simulink model "Schwingungstilger"  (R2024b)
settings: Solver=VariableStepAuto  StartTime=0.0  StopTime=10  RelTol=1e-13  AbsTol=1e-13
values from neighbouring files (symbols this model uses):
  c1 = 100e3    (= 100000)    [Schwingungstilger_Skript.m]    (also in Schwingungstilger_Skript_3d_v2.m; Schwingungstilger_Skript_fminsearch.m; v3_3d_finish.mat; v3_3d_finish_correct.mat)
  c2 = c2_man    (= 3650)    [Schwingungstilger_Skript.m]    (also in Schwingungstilger_Skript_3d_redraw_v2.m = c2_values(cIdx); Schwingungstilger_Skript_3d_v2.m = c2_values(cIdx); Schwingungstilger_Skript_fminsearch.m = params(1); v3_3d_finish.mat = 5000)
  d2 = 15    [Schwingungstilger_Skript.m]    (also in Schwingungstilger_Skript_3d_v2.m; Schwingungstilger_Skript_fminsearch.m; v3_3d_finish.mat; v3_3d_finish_correct.mat)
  m1 = 500    [Schwingungstilger_Skript.m]    (also in Schwingungstilger_Skript_3d_v2.m; Schwingungstilger_Skript_fminsearch.m; v3_3d_finish.mat; v3_3d_finish_correct.mat)
  m2 = 20    [Schwingungstilger_Skript.m]    (also in Schwingungstilger_Skript_3d_v2.m; Schwingungstilger_Skript_fminsearch.m; v3_3d_finish.mat; v3_3d_finish_correct.mat)
  x1_0 = 1    [Schwingungstilger_Skript.m]    (also in Schwingungstilger_Skript_3d_v2.m; Schwingungstilger_Skript_fminsearch.m; v3_3d_finish.mat; v3_3d_finish_correct.mat)
  x2_0 = 0    [Schwingungstilger_Skript.m]    (also in Schwingungstilger_Skript_3d_v2.m; Schwingungstilger_Skript_fminsearch.m; v3_3d_finish.mat; v3_3d_finish_correct.mat)
settings Model: Creator=phant  LastModifiedBy=msche

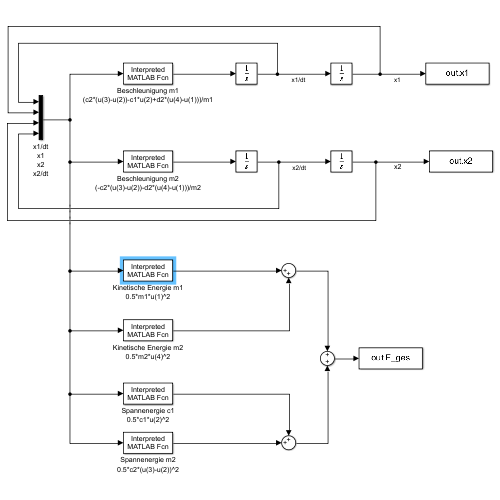
[thumbnail: Simulink's stored preview of the top-level diagram]
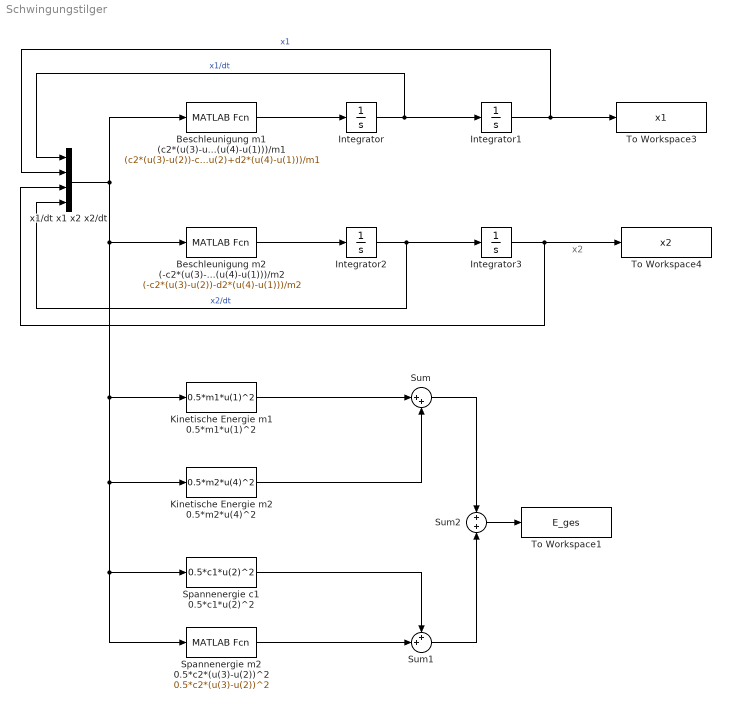
== system Schwingungstilger ==
  note: x2
  Beschleunigung m1 (c2*(u(3)-u(2))-c1*u(2)+d2*(u(4)-u(1)))/m1 : MATLABFcn  MATLABFcn=(c2*(u(3)-u(2))-c1*u(2)+d2*(u(4)-u(1)))/m1
  Beschleunigung m2 (-c2*(u(3)-u(2))-d2*(u(4)-u(1)))/m2 : MATLABFcn  MATLABFcn=(-c2*(u(3)-u(2))-d2*(u(4)-u(1)))/m2
  Integrator : Integrator
  Integrator1 : Integrator  InitialCondition=x1_0
  Integrator2 : Integrator
  Integrator3 : Integrator  InitialCondition=x2_0
  Kinetische Energie m1 0.5*m1*u(1)^2 : MATLABFcn  MATLABFcn=0.5*m1*u(1)^2
  Kinetische Energie m2 0.5*m2*u(4)^2 : MATLABFcn  MATLABFcn=0.5*m2*u(4)^2
  Spannenergie c1 0.5*c1*u(2)^2 : MATLABFcn  MATLABFcn=0.5*c1*u(2)^2
  Spannenergie m2 0.5*c2*(u(3)-u(2))^2 : MATLABFcn  MATLABFcn=0.5*c2*(u(3)-u(2))^2
  Sum : Sum  Inputs=|++
  Sum1 : Sum  Inputs=++|
  Sum2 : Sum  Inputs=+|+
  To Workspace1 : ToWorkspace  VariableName=E_ges  SaveFormat=Timeseries  SampleTime=-1
  To Workspace3 : ToWorkspace  VariableName=x1  SaveFormat=Timeseries  SampleTime=-1
  To Workspace4 : ToWorkspace  VariableName=x2  SaveFormat=Timeseries  SampleTime=-1
  x1/dt x1 x2 x2/dt : Mux
  wires:
  Integrator/1 -> x1/dt x1 x2 x2/dt/1, Integrator1/1  "x1/dt"
  Integrator1/1 -> x1/dt x1 x2 x2/dt/2, To Workspace3/1  "x1"
  Beschleunigung m1 (c2*(u(3)-u(2))-c1*u(2)+d2*(u(4)-u(1)))/m1/1 -> Integrator/1
  Integrator2/1 -> Integrator3/1, x1/dt x1 x2 x2/dt/4  "x2/dt"
  Beschleunigung m2 (-c2*(u(3)-u(2))-d2*(u(4)-u(1)))/m2/1 -> Integrator2/1
  Integrator3/1 -> To Workspace4/1, x1/dt x1 x2 x2/dt/3
  Sum/1 -> Sum2/1
  Kinetische Energie m1 0.5*m1*u(1)^2/1 -> Sum/1
  Spannenergie m2 0.5*c2*(u(3)-u(2))^2/1 -> Sum1/2
  Kinetische Energie m2 0.5*m2*u(4)^2/1 -> Sum/2
  Sum1/1 -> Sum2/2
  Sum2/1 -> To Workspace1/1
  x1/dt x1 x2 x2/dt/1 -> Beschleunigung m2 (-c2*(u(3)-u(2))-d2*(u(4)-u(1)))/m2/1, Spannenergie c1 0.5*c1*u(2)^2/1, Spannenergie m2 0.5*c2*(u(3)-u(2))^2/1, Kinetische Energie m2 0.5*m2*u(4)^2/1, Kinetische Energie m1 0.5*m1*u(1)^2/1, Beschleunigung m1 (c2*(u(3)-u(2))-c1*u(2)+d2*(u(4)-u(1)))/m1/1
  Spannenergie c1 0.5*c1*u(2)^2/1 -> Sum1/1
